simulink model "AlterPieroModelo"  (R2023b)
settings: Solver=VariableStepAuto  StartTime=0.0  StopTime=10.0  RelTol=1e-3
settings Model: Creator=Usuario_UMA  LastModifiedBy=Usuario_UMA

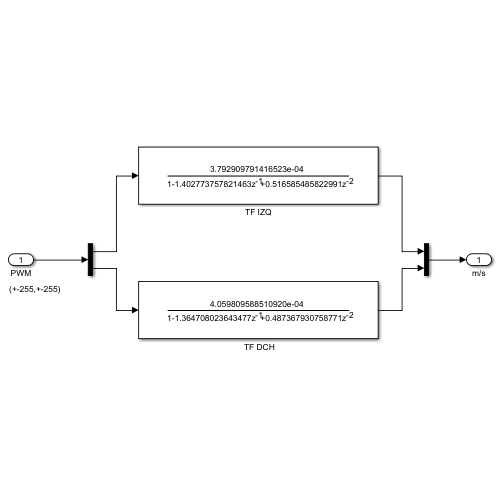
[thumbnail: Simulink's stored preview of the top-level diagram]
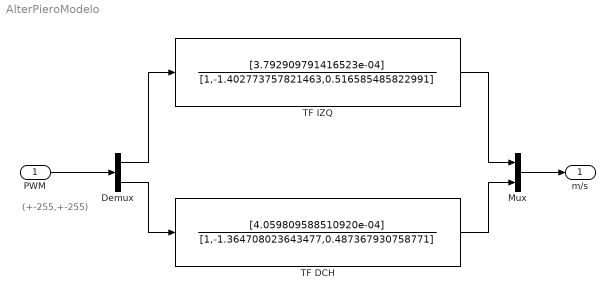
== system AlterPieroModelo ==
  note: (+-255,+-255)
  PWM : Inport
  " TF DCH" : DiscreteFilter  Numerator=[4.059809588510920e-04]  Denominator=[1,-1.364708023643477,0.487367930758771]
  Demux : Demux  Outputs=2
  Mux : Mux  Inputs=2
  TF IZQ : DiscreteFilter  Numerator=[3.792909791416523e-04]  Denominator=[1,-1.402773757821463,0.516585485822991]
  m/s : Outport
  wires:
  PWM/1 -> Demux/1
  Mux/1 -> m/s/1
  Demux/1 -> TF IZQ/1
  Demux/2 -> " TF DCH"/1
  TF IZQ/1 -> Mux/1
  " TF DCH"/1 -> Mux/2
